simulink model "simulink_model_for_the_double_spring_damper_system"  (R2024b)
settings: Solver=VariableStepAuto  StartTime=0.0  StopTime=200  RelTol=1e-3
values from neighbouring files (symbols this model uses):
  d1 = 0.5    [variables_for_parameters.m]
  d2 = 0.7    [variables_for_parameters.m]
  F = 1    [untitled.m]    (also in variables_for_parameters.m = 2)
  k1 = 10    [variables_for_parameters.m]
  k2 = 12    [variables_for_parameters.m]
  m1 = 1    [variables_for_parameters.m]
  m2 = 1.5    [variables_for_parameters.m]
  x1 = 0.2    [variables_for_parameters.m]
  x2 = 0    [variables_for_parameters.m]
  x4 = 0    [variables_for_parameters.m]
settings Model: Creator=kavin  LastModifiedBy=kavin

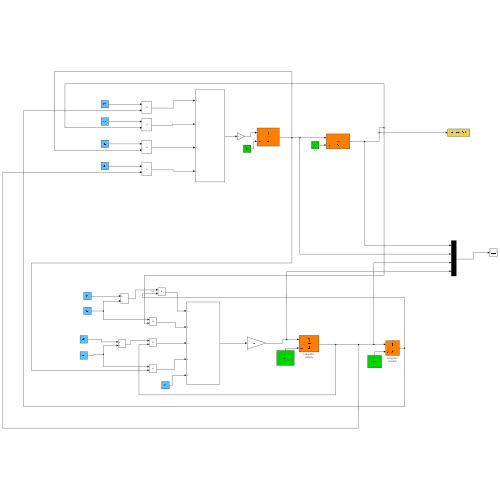
[thumbnail: Simulink's stored preview of the top-level diagram]
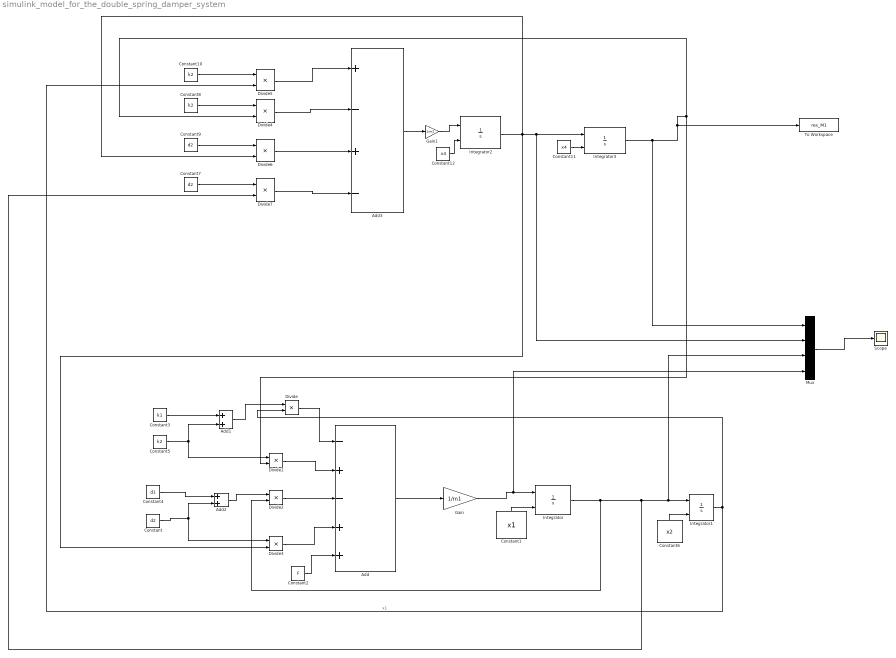
== system simulink_model_for_the_double_spring_damper_system ==
  Add : Sum  Inputs=-+-++
  Add1 : Sum
  Add2 : Sum
  Add3 : Sum  Inputs=+-+-
  Constant : Constant  Value=d2
  Constant1 : Constant  Value=x1
  Constant10 : Constant  Value=k2
  Constant11 : Constant  Value=x4
  Constant12 : Constant  Value=x4
  Constant2 : Constant  Value=F
  Constant3 : Constant  Value=k1
  Constant4 : Constant  Value=d1
  Constant5 : Constant  Value=k2
  Constant6 : Constant  Value=x2
  Constant7 : Constant  Value=d2
  Constant8 : Constant  Value=k2
  Constant9 : Constant  Value=d2
  Divide{,1..7} (8 alike) : Product  Inputs=**
  Gain : Gain  Gain=1/m1
  Gain1 : Gain  Gain=1/m2
  Integrator{,1..3} (4 alike) : Integrator  InitialConditionSource=external
      Integrator settings: AttributesFormatString=|
      | %<BlockType>
      | velocity
      Integrator1 settings: AttributesFormatString=|
      | %<BlockType>
      | position
  Mux : Mux
  Scope : Scope
  To Workspace : ToWorkspace  VariableName=res_M1  SaveFormat=Timeseries  SampleTime=-1
  wires:
  Gain/1 -> Mux/4, Integrator/1
  Add/1 -> Gain/1
  Constant/1 -> Add2/2, Divide3/1
  Constant4/1 -> Add2/1
  Constant5/1 -> Add1/2, Divide1/1
  Constant3/1 -> Add1/1
  Add2/1 -> Divide2/1
  Constant2/1 -> Add/5
  Add1/1 -> Divide/1
  Divide/1 -> Add/1
  Integrator2/1 -> Divide6/2, Mux/2, Integrator3/1, Divide3/2
  Divide1/1 -> Add/2
  Divide2/1 -> Add/3
  Divide3/1 -> Add/4
  Constant1/1 -> Integrator/2
  Constant6/1 -> Integrator1/2
  Integrator1/1 -> Divide/2, Divide5/2  "x1"
  Constant10/1 -> Divide5/1
  Constant9/1 -> Divide6/1
  Constant8/1 -> Divide4/1
  Divide4/1 -> Add3/2
  Constant7/1 -> Divide7/1
  Divide5/1 -> Add3/1
  Divide6/1 -> Add3/3
  Divide7/1 -> Add3/4
  Gain1/1 -> Integrator2/1
  Add3/1 -> Gain1/1
  Integrator3/1 -> Mux/1, Divide1/2, Divide4/2, To Workspace/1
  Constant12/1 -> Integrator2/2
  Constant11/1 -> Integrator3/2
  Mux/1 -> Scope/1
  Integrator/1 -> Divide7/2, Mux/3, Integrator1/1, Divide2/2
